simulink model "GPSNoiseModel"  (R2023a)
settings: Solver=VariableStepAuto  StartTime=0.0  StopTime=10  RelTol=1e-3
libraries: sensorgpslib x1
settings Model: Creator=The MathWorks, Inc.  LastModifiedBy=The MathWorks, Inc.
settings DebuggingCC: UnconnectedInputMsg=warning  UnconnectedOutputMsg=warning  UnconnectedLineMsg=warning
settings ModelReferenceCC: EnableRefExpFcnMdlSchedulingChecks=on
settings RTWCC: DLArmComputeVersion=19.05

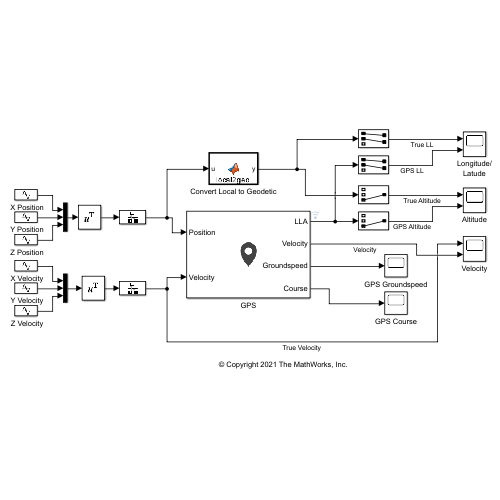
[thumbnail: Simulink's stored preview of the top-level diagram]
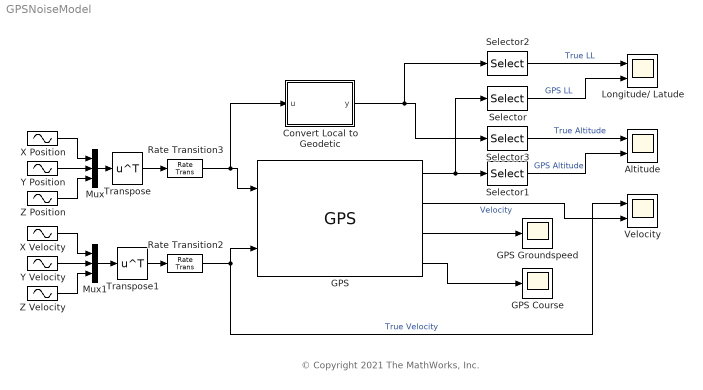
== system GPSNoiseModel ==
  note: © Copyright 2021 The MathWorks, Inc.
  " X Position" : Sin  Amplitude=3  Bias=4  Frequency=pi  SampleTime=0
  " X Velocity" : Sin  Bias=3  SampleTime=0
  " Y Position" : Sin  Amplitude=3  Frequency=pi  SampleTime=0
  " Y Velocity" : Sin  SampleTime=0
  " Z Position" : Sin  Amplitude=3  SampleTime=0
  " Z Velocity" : Sin  Bias=-3  SampleTime=0
  Altitude : Scope  NumInputPorts=2
  Convert Local to Geodetic : MATLAB Function  TreatAsAtomicUnit=on
  GPS : sensorgpslib/GPS  DispRefFrame=NED  PositionInputFormat=Local  ReferenceLocation=[ 0, 0, 0 ]  HorizontalPositionAccuracy=1.6  VerticalPositionAccuracy=.5  VelocityAccuracy=0.1  DecayFactor=0.999  SeedDouble=67  SimulateUsing=Interpreted execution
  GPS Course : Scope
  GPS Groundspeed : Scope
  Longitude/ Latude : Scope  NumInputPorts=2
  Mux : Mux  Inputs=3
  Mux1 : Mux  Inputs=3
  Rate Transition2 : RateTransition  OutPortSampleTime=.01
  Rate Transition3 : RateTransition  OutPortSampleTime=.01
  Selector : Selector  InputPortWidth=3  IndexOptions=Index vector (dialog)  Indices=[1 2]  OutputSizes=1
  Selector1 : Selector  InputPortWidth=3  IndexOptions=Index vector (dialog)  Indices=[3]  OutputSizes=1
  Selector2 : Selector  InputPortWidth=3  IndexOptions=Index vector (dialog)  Indices=[1 2]  OutputSizes=1
  Selector3 : Selector  InputPortWidth=3  IndexOptions=Index vector (dialog)  Indices=[3]  OutputSizes=1
  Transpose : Math  Operator=transpose
  Transpose1 : Math  Operator=transpose
  Velocity : Scope  NumInputPorts=2
  wires:
  GPS/2 -> Velocity/2  "Velocity"
  GPS/3 -> GPS Groundspeed/1
  GPS/4 -> GPS Course/1
  GPS/1 -> Selector/1, Selector1/1
  " X Position"/1 -> Mux/1
  Mux/1 -> Transpose/1
  " Y Position"/1 -> Mux/2
  " Z Position"/1 -> Mux/3
  " X Velocity"/1 -> Mux1/1
  " Y Velocity"/1 -> Mux1/2
  " Z Velocity"/1 -> Mux1/3
  Mux1/1 -> Transpose1/1
  Transpose1/1 -> Rate Transition2/1
  Rate Transition2/1 -> Velocity/1, GPS/2  "True Velocity"
  Transpose/1 -> Rate Transition3/1
  Rate Transition3/1 -> Convert Local to Geodetic/1(u), GPS/1
  Convert Local to Geodetic/1(y) -> Selector3/1, Selector2/1
  Selector/1 -> Longitude/ Latude/2  "GPS LL"
  Selector2/1 -> Longitude/ Latude/1  "True LL"
  Selector3/1 -> Altitude/1  "True Altitude"
  Selector1/1 -> Altitude/2  "GPS Altitude"

== matlab function GPSNoiseModel/Convert Local to Geodetic ==
  data: u input; y output
function y = local2geo(u)

y = ned2lla(u,[0 0 0],"ellipsoid");

end
